simulink subsystem "Goal_Subsystem"  (R2022b)
settings: Solver=VariableStepAuto  StartTime=0.0  StopTime=10.0  RelTol=1e-3
settings Model: Creator=ROG  LastModifiedBy=Sahil Gaurkar

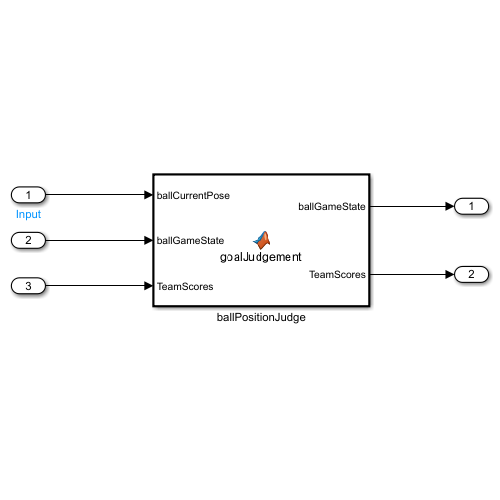
[thumbnail: Simulink's stored preview of the top-level diagram]
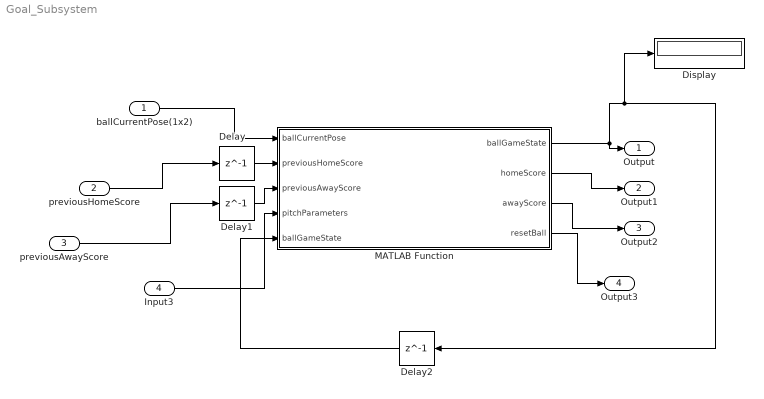
== system Goal_Subsystem ==
  ballCurrentPose(1x2) : Inport
  previousHomeScore : Inport  Port=2
  previousAwayScore : Inport  Port=3
  Input3 : Inport  Port=4
  Delay : Delay  DelayLength=1
  Delay1 : Delay  DelayLength=1
  Delay2 : Delay  DelayLength=1
  Display : Display
  MATLAB Function : MATLAB Function  TreatAsAtomicUnit=on
  Output : Outport
  Output1 : Outport  Port=2
  Output2 : Outport  Port=3
  Output3 : Outport  Port=4
  wires:
  Delay2/1 -> MATLAB Function/5("ballGameState ")
  Delay1/1 -> MATLAB Function/3(previousAwayScore)
  Delay/1 -> MATLAB Function/2(previousHomeScore)
  previousAwayScore/1 -> Delay1/1
  ballCurrentPose(1x2)/1 -> MATLAB Function/1(ballCurrentPose)
  previousHomeScore/1 -> Delay/1
  MATLAB Function/2(homeScore) -> Output1/1
  MATLAB Function/1(ballGameState) -> Delay2/1, Display/1, Output/1
  MATLAB Function/3(awayScore) -> Output2/1
  Input3/1 -> MATLAB Function/4(pitchParameters)
  MATLAB Function/4(resetBall) -> Output3/1

== matlab function Goal_Subsystem/MATLAB Function ==
  data: ballCurrentPose input; ballGameState output; previousHomeScore input; previousAwayScore input; pitchParameters input; homeScore output double size=1; awayScore output double size=1; ballGameState input; resetBall output
function [ballGameState,homeScore, awayScore, resetBall] = goalJudgement(ballCurrentPose, previousHomeScore, previousAwayScore, pitchParameters, ballGameState)
%     gameState : 0->normal, 1->scored ,2->out of boundary,

    resetBall = 0;

%     Depart Team Score
    homeScore = previousHomeScore;
    awayScore = previousAwayScore;

%     get ball X, Y 
    ballCurrentX = ballCurrentPose(1);
    ballCurrentY = ballCurrentPose(2);
    
    if (ballGameState == 1 || ballGameState == 2)

        ballGameState = 0;

    elseif (ballCurrentX < (-pitchParameters(1)/2) && ballCurrentY > -pitchParameters(9)/2 && ballCurrentY <  pitchParameters(9)/2)
        % Away Team scored
        % Away Team socre + 1
        awayScore = awayScore + 1;
        ballGameState = 1;
        resetBall = 1;
       
    elseif (ballCurrentX >= (pitchParameters(1)/2) && ballCurrentY > -pitchParameters(9)/2 && ballCurrentY < pitchParameters(9)/2)
        % Our Team scored
        % Our Team socre + 1
        homeScore = homeScore + 1;
        ballGameState = 1;
        resetBall = 1;

    end

    if ballGameState == 0
        if ((ballCurrentY > pitchParameters(2)/2) || ballCurrentY < (-pitchParameters(2)/2)) || (ballCurrentX > (pitchParameters(1)/2) || ballCurrentX < (-pitchParameters(1)/2))
            ballGameState = 2; % 5 is ball out of bounds state
            resetBall = 1;
        end
    end


%     if ballGameState == 1
%         % normal play
%     end    
end
